simulink model "identMF"  (R2014a)
settings: Solver=ode45  StartTime=0.0  StopTime=20  MaxStep=0.01  RelTol=1e-3
settings Model: Creator=Bruno  LastModifiedBy=Luiz Carlos
settings DataIOCC: SignalLoggingSaveFormat=ModelDataLogs
settings OptimizationCC: ExpressionDepthLimit=2147483647
settings DebuggingCC: UnderspecifiedInitializationDetection=Classic  FcnCallInpInsideContextMsg=UseLocalSettings  StateNameClashWarn=warning
settings GRTTargetCC: CombineOutputUpdateFcns=off  GRTInterface=on

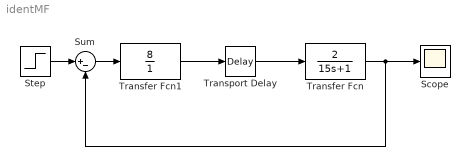
== system identMF ==
  Scope : Scope
      settings: TimeRange=4.335126825518832  YMin=0.9237500000000001  YMax=1.06875
  Step : Step  SampleTime=0
  Sum : Sum  Inputs=|+-
  Transfer Fcn : TransferFcn  Numerator=[2]  Denominator=[15 1]
  Transfer Fcn1 : TransferFcn  Numerator=[8]  Denominator=[1]
  Transport Delay : TransportDelay
  wires:
  Sum/1 -> Transfer Fcn1/1
  Transfer Fcn1/1 -> Transport Delay/1
  Transport Delay/1 -> Transfer Fcn/1
  Transfer Fcn/1 -> Sum/2, Scope/1
  Step/1 -> Sum/1
